simulink model "hyd_hyb_2_int_cont_offline"  (Simulink 8.2)
settings: Solver=ode4  StartTime=0  StopTime=560  FixedStep=0.01  MaxStep=.4  RelTol=1e-8
InitFcn:
  | const_3
values from neighbouring files (symbols this model uses):
  Af = 6.3    [brk_enrg.m]    (also in brk_enrg_1.m)
  BSFC_906_205 = [3.5684 4.3466 5.1668 6.0769 6.988 7.8992 8.8104 9.7336 10.8548 11.9809 13.1112 14.2571 ... (663 elements, 39x17)]    [BSFC_map_906_205.mat]
  Cd = 0.55    [brk_enrg.m]    (also in brk_enrg_1.m)
  den = 1.202    [brk_enrg.m]    (also in brk_enrg_1.m)
  fr = 0.01    [brk_enrg.m]    (also in brk_enrg_1.m)
undefined symbols (not defined in the file or in its folder): clutchRise, down_spd_2, down_spd_3, down_spd_4, down_spd_c, fuel_density, gearshift, I_wheel, Idle_spd_eng_906, M1_hydr, p_v_15, pmax_125, qv_125, Rw, sec_eng_sfc_map, T_max_906, T_min, TC_spd_ratio_max, torque_convertor, Twait, up_spd_1, up_spd_2, up_spd_3, up_spd_c, v_p_10, v_p_15, v_p_5
libraries: fl_lib x43, nesl_utility x30, sdl_lib x14, simulink x4, simulink_need_slupdate x1
(part 2 of 3)

== system hyd_hyb_2_int_cont_offline/hydraulic transmission/controller ==
  T_error : Inport
  Gain : Gain  Gain=1.4
  PID Controller : simulink_need_slupdate/PID Controller  P=0.1  I=10  D=0
  Saturation : Saturate  UpperLimit=125  LowerLimit=-125
  Scope : Scope
      settings: YMin=0  YMax=105  SaveName=ScopeData5
  Transfer Fcn : TransferFcn  Numerator=[1 0]  Denominator=[1 5]
  vg(cm^3/rev) : Outport
  wires:
  T_error/1 -> Gain/1
  Gain/1 -> PID Controller/1
  Saturation/1 -> vg(cm^3/rev)/1
  PID Controller/1 -> Transfer Fcn/1
  Transfer Fcn/1 -> Saturation/1

== system hyd_hyb_2_int_cont_offline/post-transmission torque coupling/Sensor(coupling) ==
  Motion sensor : Subsystem
  Torque sensor : Subsystem
  A : PMIOPort  Port=1  Side=Left
  B : PMIOPort  Port=2  Side=Right
  tag scope: T_coupling=global, w_coupling=global
  wires:
  Torque sensor/1(T) -> [T_coupling]
  Motion sensor/1(W) -> [w_coupling]
  connections:
  B/RConn1 -- Torque sensor/RConn1
  Torque sensor/LConn1 -- Motion sensor/LConn1 -- A/RConn1

== system hyd_hyb_2_int_cont_offline/post-transmission torque coupling/pm gearbox ==
  Ideal Torque Sensor : fl_lib/Mechanical/Mechanical Sensors/Ideal Torque Sensor  w_Log=off  t_Log=off  LocalVarNames=|w|t  LocalVarDescs=|w|t  LocalVarLogging=[0 0]
  Memory : Memory
  PS-Simulink Converter : nesl_utility/PS-Simulink Converter  PhysicalDomain=network_engine_domain  SubClassName=ps_output  LeftPortType=input  RightPortType=output  PseudoPeriodic=off  Frequencies=[]  Unit=N*m  AffineConversion=off
  Simple Gear1 : sdl_lib/Gears/Simple Gear  ratio=1.75  rotation_direction=1  friction_model=1  T_noload=0.1 N*m  T_nom=5 N*m  efficiency_nom=0.8  efficiency=0.8  mu_visc=[ 0 0 ] N*m/(rad/s)  w_thr=0.01 rad/s  LocalVarLogging=[]
  Connection Port : PMIOPort  Tag=PMCPort  Port=1  Side=Left
  Connection Port1 : PMIOPort  Tag=PMCPort  Port=2  Side=Right
  P/M actu_torq(N.m) : Outport
  wires:
  Memory/1 -> P/M actu_torq(N.m)/1
  PS-Simulink Converter/1 -> Memory/1
  connections:
  Simple Gear1/LConn1 -- Connection Port/RConn1
  Simple Gear1/RConn1 -- Ideal Torque Sensor/LConn1
  Ideal Torque Sensor/RConn1 -- Connection Port1/RConn1
  Ideal Torque Sensor/RConn2 -- PS-Simulink Converter/LConn1

== system hyd_hyb_2_int_cont_offline/Engine/Consumption Calc (nmap)1/sfc corrector ==
  main map : Inport
  eng_spd(rpm) : Inport  Port=2
  eng_pow(kw) : Inport  Port=3
  Constant : Constant  Value=Idle_spd_eng_906
  Constant1 : Constant  Value=1000
  Gain : Gain  Gain=-1
  Gain1 : Gain
  Gain2 : Gain
  Product : Product  Inputs=*/  RndMeth=Zero
  Product1 : Product  Inputs=*/  RndMeth=Zero
  Product2 : Product  RndMeth=Zero
  Product3 : Product  RndMeth=Zero
  Scope : Scope  NumInputPorts=2
      settings: YMin=-5~-5  YMax=5~5  SaveName=ScopeData40
  Scope1 : Scope  NumInputPorts=2
      settings: YMin=-5~-5  YMax=5~5  SaveName=ScopeData41
  Scope2 : Scope  NumInputPorts=2
      settings: YMin=-5~-5  YMax=5~5  SaveName=ScopeData42
  Sum : Sum  Inputs=|+-
  Sum1 : Sum  Inputs=|+-
  Sum2 : Sum  Inputs=|+-
  Sum3 : Sum  Inputs=|++
  Switch : Switch  Threshold=1000
  sec_eng_sfc_map (906) : Lookup  InputValues=sec_eng_sfc_map(:,1)  Table=sec_eng_sfc_map(:,2)
  cons(kg/h) : Outport
  wires:
  Gain2/1 -> Product2/1, Scope2/2
  eng_pow(kw)/1 -> sec_eng_sfc_map (906)/1
  Switch/1 -> cons(kg/h)/1
  Sum3/1 -> Switch/3, Scope/2
  Product3/1 -> Sum3/2, Scope1/2
  Product2/1 -> Sum3/1, Scope1/1
  main map/1 -> Product3/1, Switch/1, Scope/1
  sec_eng_sfc_map (906)/1 -> Gain2/1, Scope2/1
  Product1/1 -> Product3/2  "b"
  Gain1/1 -> Product1/1
  Sum2/1 -> Gain1/1
  Product/1 -> Product2/2  "a"
  Sum1/1 -> Product1/2, Product/2
  Constant/1 -> Sum2/2, Sum1/2
  Gain/1 -> Product/1
  Sum/1 -> Gain/1
  Constant1/1 -> Sum1/1, Sum/2
  eng_spd(rpm)/1 -> Switch/2, Sum2/1, Sum/1

== system hyd_hyb_2_int_cont_offline/Engine/Sensor(eng)/Motion sensor ==
  Ideal Rotational Motion Sensor : fl_lib/Mechanical/Mechanical Sensors/Ideal Rotational Motion Sensor  offset=0 rad  w_Log=off  t_Log=off  phi_Log=off  LocalVarNames=|w|t|phi  LocalVarDescs=|w|t|phi  LocalVarLogging=[]
  MRR : fl_lib/Mechanical/Rotational Elements/Mechanical Rotational Reference  t_Log=off  LocalVarNames=|t  LocalVarDescs=|t  LocalVarLogging=[]
  PS-Simulink Converter : nesl_utility/PS-Simulink Converter  PhysicalDomain=network_engine_domain  SubClassName=ps_output  LeftPortType=input  RightPortType=output  PseudoPeriodic=off  Frequencies=[]  Unit=rad/s  AffineConversion=off
  A : PMIOPort  Port=1  Side=Left
  W : Outport
  wires:
  PS-Simulink Converter/1 -> W/1
  connections:
  MRR/LConn1 -- Ideal Rotational Motion Sensor/RConn1
  Ideal Rotational Motion Sensor/RConn2 -- PS-Simulink Converter/LConn1
  A/RConn1 -- Ideal Rotational Motion Sensor/LConn1

== system hyd_hyb_2_int_cont_offline/Engine/Sensor(eng)/Torque sensor ==
  PS2S : nesl_utility/PS-Simulink Converter  PhysicalDomain=network_engine_domain  SubClassName=ps_output  LeftPortType=input  RightPortType=output  PseudoPeriodic=off  Frequencies=[]  Unit=1  AffineConversion=off
  Torque Sensor : fl_lib/Mechanical/Mechanical Sensors/Ideal Torque Sensor  w_Log=off  t_Log=off  LocalVarNames=|w|t  LocalVarDescs=|w|t  LocalVarLogging=[]
  B : PMIOPort  Port=1  Side=Right
  A : PMIOPort  Port=2  Side=Left
  T : Outport
  wires:
  PS2S/1 -> T/1
  connections:
  Torque Sensor/RConn2 -- PS2S/LConn1
  B/RConn1 -- Torque Sensor/RConn1
  A/RConn1 -- Torque Sensor/LConn1

== system hyd_hyb_2_int_cont_offline/Transmission1/Sensor(GB_out)/Motion sensor ==
  Ideal Rotational Motion Sensor : fl_lib/Mechanical/Mechanical Sensors/Ideal Rotational Motion Sensor  offset=0 rad  w_Log=off  t_Log=off  phi_Log=off  LocalVarNames=|w|t|phi  LocalVarDescs=|w|t|phi  LocalVarLogging=[]
  MRR : fl_lib/Mechanical/Rotational Elements/Mechanical Rotational Reference  t_Log=off  LocalVarNames=|t  LocalVarDescs=|t  LocalVarLogging=[]
  PS-Simulink Converter : nesl_utility/PS-Simulink Converter  PhysicalDomain=network_engine_domain  SubClassName=ps_output  LeftPortType=input  RightPortType=output  PseudoPeriodic=off  Frequencies=[]  Unit=rad/s  AffineConversion=off
  A : PMIOPort  Port=1  Side=Left
  W : Outport
  wires:
  PS-Simulink Converter/1 -> W/1
  connections:
  A/RConn1 -- Ideal Rotational Motion Sensor/LConn1
  Ideal Rotational Motion Sensor/RConn2 -- PS-Simulink Converter/LConn1
  MRR/LConn1 -- Ideal Rotational Motion Sensor/RConn1

== system hyd_hyb_2_int_cont_offline/Transmission1/Sensor(GB_out)/Torque sensor ==
  PS2S : nesl_utility/PS-Simulink Converter  PhysicalDomain=network_engine_domain  SubClassName=ps_output  LeftPortType=input  RightPortType=output  PseudoPeriodic=off  Frequencies=[]  Unit=1  AffineConversion=off
  Torque Sensor : fl_lib/Mechanical/Mechanical Sensors/Ideal Torque Sensor  w_Log=off  t_Log=off  LocalVarNames=|w|t  LocalVarDescs=|w|t  LocalVarLogging=[]
  B : PMIOPort  Port=1  Side=Right
  A : PMIOPort  Port=2  Side=Left
  T : Outport
  wires:
  PS2S/1 -> T/1
  connections:
  A/RConn1 -- Torque Sensor/LConn1
  B/RConn1 -- Torque Sensor/RConn1
  Torque Sensor/RConn2 -- PS2S/LConn1

== system hyd_hyb_2_int_cont_offline/Transmission1/Sensor(TC_GB)/Motion sensor ==
  Ideal Rotational Motion Sensor : fl_lib/Mechanical/Mechanical Sensors/Ideal Rotational Motion Sensor  offset=0 rad  w_Log=off  t_Log=off  phi_Log=off  LocalVarNames=|w|t|phi  LocalVarDescs=|w|t|phi  LocalVarLogging=[]
  MRR : fl_lib/Mechanical/Rotational Elements/Mechanical Rotational Reference  t_Log=off  LocalVarNames=|t  LocalVarDescs=|t  LocalVarLogging=[]
  PS-Simulink Converter : nesl_utility/PS-Simulink Converter  PhysicalDomain=network_engine_domain  SubClassName=ps_output  LeftPortType=input  RightPortType=output  PseudoPeriodic=off  Frequencies=[]  Unit=rad/s  AffineConversion=off
  A : PMIOPort  Port=1  Side=Left
  W : Outport
  wires:
  PS-Simulink Converter/1 -> W/1
  connections:
  MRR/LConn1 -- Ideal Rotational Motion Sensor/RConn1
  Ideal Rotational Motion Sensor/RConn2 -- PS-Simulink Converter/LConn1
  A/RConn1 -- Ideal Rotational Motion Sensor/LConn1

== system hyd_hyb_2_int_cont_offline/Transmission1/Sensor(TC_GB)/Torque sensor ==
  PS2S : nesl_utility/PS-Simulink Converter  PhysicalDomain=network_engine_domain  SubClassName=ps_output  LeftPortType=input  RightPortType=output  PseudoPeriodic=off  Frequencies=[]  Unit=1  AffineConversion=off
  Torque Sensor : fl_lib/Mechanical/Mechanical Sensors/Ideal Torque Sensor  w_Log=off  t_Log=off  LocalVarNames=|w|t  LocalVarDescs=|w|t  LocalVarLogging=[]
  B : PMIOPort  Port=1  Side=Right
  A : PMIOPort  Port=2  Side=Left
  T : Outport
  wires:
  PS2S/1 -> T/1
  connections:
  Torque Sensor/RConn2 -- PS2S/LConn1
  B/RConn1 -- Torque Sensor/RConn1
  A/RConn1 -- Torque Sensor/LConn1

== system hyd_hyb_2_int_cont_offline/Transmission1/Torque Convertor/main solver ==
  Add : Sum  Inputs=+-
  Ideal Torque Source1 : fl_lib/Mechanical/Mechanical Sources/Ideal Torque Source  w_Log=off  t_Log=off  LocalVarNames=|w|t  LocalVarDescs=|w|t  LocalVarLogging=[0 0]
  Ideal Torque Source2 : fl_lib/Mechanical/Mechanical Sources/Ideal Torque Source  w_Log=off  t_Log=off  LocalVarNames=|w|t  LocalVarDescs=|w|t  LocalVarLogging=[0 0]
  Mechanical Rotational Reference1 : fl_lib/Mechanical/Rotational Elements/Mechanical Rotational Reference  t_Log=off  LocalVarNames=|t  LocalVarDescs=|t  LocalVarLogging=0
  Sensor(TC_in) : Subsystem
  Sensor(TC_out) : Subsystem
  Simulink-PS Converter1 : nesl_utility/Simulink-PS Converter  PhysicalDomain=network_engine_domain  SubClassName=ps_input  LeftPortType=input  RightPortType=output  PseudoPeriodic=off  Frequencies=[]  NoiseDistribution=none  NoiseParameters=[]  Unit=1  AffineConversion=off  InputFiltering=off  SimscapeFilterOrder=1  InputFilterTimeConstant=0.01  UdotUserProvided=0
  Simulink-PS Converter2 : nesl_utility/Simulink-PS Converter  PhysicalDomain=network_engine_domain  SubClassName=ps_input  LeftPortType=input  RightPortType=output  PseudoPeriodic=off  Frequencies=[]  NoiseDistribution=none  NoiseParameters=[]  Unit=1  AffineConversion=off  InputFiltering=off  SimscapeFilterOrder=1  InputFilterTimeConstant=0.01  UdotUserProvided=0
  Torque generation : Subsystem  AncestorBlock=|
      | driveline/Dynamic
      | Elements/Torque
      | Converter/Torque generation
  T : PMIOPort  Tag=PMCPort  Port=1  Side=Right
  I : PMIOPort  Tag=PMCPort  Port=2  Side=Left
  Turbine torque : Outport
  wires:
  [w_TC_in] -> Torque generation/2(Impeller speed (rad/s))
  Torque generation/1(Turbine torque) -> Turbine torque/1, Simulink-PS Converter1/1
  [w_TC_out] -> Torque generation/1(Turbine speed (rad/s))
  Torque generation/2(Impeller torque) -> Add/1
  [Aux_Trq] -> Add/2
  Add/1 -> Simulink-PS Converter2/1
  connections:
  Ideal Torque Source2/RConn2 -- Mechanical Rotational Reference1/LConn1 -- Ideal Torque Source1/RConn2
  Simulink-PS Converter1/RConn1 -- Ideal Torque Source1/RConn1
  Ideal Torque Source2/RConn1 -- Simulink-PS Converter2/RConn1
  Ideal Torque Source1/LConn1 -- Sensor(TC_out)/LConn1
  Sensor(TC_out)/RConn1 -- T/RConn1
  Ideal Torque Source2/LConn1 -- Sensor(TC_in)/LConn1
  Sensor(TC_in)/RConn1 -- I/RConn1

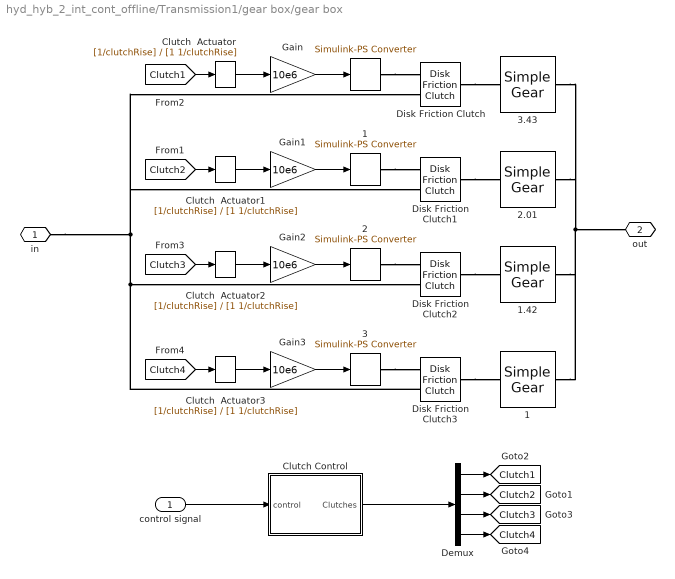
== system hyd_hyb_2_int_cont_offline/Transmission1/gear box/gear box ==
  control signal : Inport
   {,1..3} (4 alike) : nesl_utility/Simulink-PS Converter  PhysicalDomain=network_engine_domain  SubClassName=ps_input  LeftPortType=input  RightPortType=output  PseudoPeriodic=off  Frequencies=[]  NoiseDistribution=none  NoiseParameters=[]  Unit=1  AffineConversion=off  InputFiltering=off  SimscapeFilterOrder=1  InputFilterTimeConstant=0.01  UdotUserProvided=0
  1 : sdl_lib/Gears/Simple Gear  ratio=1  rotation_direction=1  friction_model=1  T_noload=0.1 N*m  T_nom=5 N*m  efficiency_nom=0.8  efficiency=0.8  mu_visc=[ 0 0 ] N*m/(rad/s)  w_thr=0.01 rad/s  LocalVarLogging=[]
  1.42 : sdl_lib/Gears/Simple Gear  ratio=1.42  rotation_direction=1  friction_model=1  T_noload=0.1 N*m  T_nom=5 N*m  efficiency_nom=0.8  efficiency=0.8  mu_visc=[ 0 0 ] N*m/(rad/s)  w_thr=0.01 rad/s  LocalVarLogging=[]
  2.01 : sdl_lib/Gears/Simple Gear  ratio=2.01  rotation_direction=1  friction_model=1  T_noload=0.1 N*m  T_nom=5 N*m  efficiency_nom=0.8  efficiency=0.8  mu_visc=[ 0 0 ] N*m/(rad/s)  w_thr=0.01 rad/s  LocalVarLogging=[]
  3.43 : sdl_lib/Gears/Simple Gear  ratio=3.43  rotation_direction=1  friction_model=1  T_noload=0.1 N*m  T_nom=5 N*m  efficiency_nom=0.8  efficiency=0.8  mu_visc=[ 0 0 ] N*m/(rad/s)  w_thr=0.01 rad/s  LocalVarLogging=[]
  Clutch  Actuator{,1..3} (4 alike) : TransferFcn  Numerator=[1/clutchRise]  Denominator=[1 1/clutchRise]
  Clutch Control : Subsystem
  Demux : Demux
  Disk Friction Clutch : sdl_lib/Clutches/Disk Friction Clutch  geometry_model=1  r_eff=1 m  d_o=150 mm  d_i=100 mm  nS=8  piston_area=0.001 m^2  friction_model=1  mu_coulomb=0.3  mu_w_vector=[ 0 0.1 0.2 0.3 0.4 0.5 1 2 5 10 100 1000 ] rad/s  mu_coulomb_vector=[ 0.29 0.28 0.26 0.22 0.21 0.2 0.2 0.19 0.19 0.19 0.19 0.19 ]  mu_interp_method=1  mu_extrap_method=1  mu_static=0.35  d_f=1  w_tol=0.001 rad/s  pressure_min=100 Pa  mu_visc=0 N*m/(rad/s)  initial_state_locked=0  LocalVarLogging=[]
  Disk Friction Clutch1 : sdl_lib/Clutches/Disk Friction Clutch  geometry_model=1  r_eff=.1 m  d_o=150 mm  d_i=100 mm  nS=8  piston_area=0.001 m^2  friction_model=1  mu_coulomb=0.3  mu_w_vector=[ 0 0.1 0.2 0.3 0.4 0.5 1 2 5 10 100 1000 ] rad/s  mu_coulomb_vector=[ 0.29 0.28 0.26 0.22 0.21 0.2 0.2 0.19 0.19 0.19 0.19 0.19 ]  mu_interp_method=1  mu_extrap_method=1  mu_static=0.35  d_f=1  w_tol=0.001 rad/s  pressure_min=100 Pa  mu_visc=0 N*m/(rad/s)  initial_state_locked=0  LocalVarLogging=[]
  Disk Friction Clutch2 : sdl_lib/Clutches/Disk Friction Clutch  geometry_model=1  r_eff=1 m  d_o=150 mm  d_i=100 mm  nS=8  piston_area=0.001 m^2  friction_model=1  mu_coulomb=0.3  mu_w_vector=[ 0 0.1 0.2 0.3 0.4 0.5 1 2 5 10 100 1000 ] rad/s  mu_coulomb_vector=[ 0.29 0.28 0.26 0.22 0.21 0.2 0.2 0.19 0.19 0.19 0.19 0.19 ]  mu_interp_method=1  mu_extrap_method=1  mu_static=0.35  d_f=1  w_tol=0.001 rad/s  pressure_min=100 Pa  mu_visc=0 N*m/(rad/s)  initial_state_locked=0  LocalVarLogging=[]
  Disk Friction Clutch3 : sdl_lib/Clutches/Disk Friction Clutch  geometry_model=1  r_eff=1 m  d_o=150 mm  d_i=100 mm  nS=8  piston_area=0.001 m^2  friction_model=1  mu_coulomb=0.3  mu_w_vector=[ 0 0.1 0.2 0.3 0.4 0.5 1 2 5 10 100 1000 ] rad/s  mu_coulomb_vector=[ 0.29 0.28 0.26 0.22 0.21 0.2 0.2 0.19 0.19 0.19 0.19 0.19 ]  mu_interp_method=1  mu_extrap_method=1  mu_static=0.35  d_f=1  w_tol=0.001 rad/s  pressure_min=100 Pa  mu_visc=0 N*m/(rad/s)  initial_state_locked=0  LocalVarLogging=[]
  Gain{,1..3} (4 alike) : Gain  Gain=10e6
  in : PMIOPort  Port=1  Side=Left
  out : PMIOPort  Port=2  Side=Right
  tag scope: Clutch1=global, Clutch2=global, Clutch3=global, Clutch4=global
  wires:
  control signal/1 -> Clutch Control/1(control)
  Clutch Control/1(Clutches) -> Demux/1
  Demux/1 -> [Clutch1]
  Demux/2 -> [Clutch2]
  Demux/3 -> [Clutch3]
  Demux/4 -> [Clutch4]
  [Clutch1] -> Clutch  Actuator/1
  [Clutch2] -> Clutch  Actuator1/1
  [Clutch3] -> Clutch  Actuator2/1
  [Clutch4] -> Clutch  Actuator3/1
  Clutch  Actuator/1 -> Gain/1
  Clutch  Actuator1/1 -> Gain1/1
  Clutch  Actuator2/1 -> Gain2/1
  Clutch  Actuator3/1 -> Gain3/1
  Gain/1 -> " "/1
  Gain1/1 -> " 1"/1
  Gain2/1 -> " 2"/1
  Gain3/1 -> " 3"/1
  connections:
  Disk Friction Clutch3/LConn2 -- in/RConn1 -- Disk Friction Clutch/LConn2 -- Disk Friction Clutch1/LConn2 -- Disk Friction Clutch2/LConn2
  1.42/RConn1 -- 3.43/RConn1 -- 1/RConn1 -- 2.01/RConn1 -- out/RConn1
  " "/RConn1 -- Disk Friction Clutch/LConn1
  " 1"/RConn1 -- Disk Friction Clutch1/LConn1
  " 2"/RConn1 -- Disk Friction Clutch2/LConn1
  " 3"/RConn1 -- Disk Friction Clutch3/LConn1
  Disk Friction Clutch/RConn1 -- 3.43/LConn1
  Disk Friction Clutch1/RConn1 -- 2.01/LConn1
  Disk Friction Clutch2/RConn1 -- 1.42/LConn1
  Disk Friction Clutch3/RConn1 -- 1/LConn1

== system hyd_hyb_2_int_cont_offline/Vehicle Dynamic/Resistance Load/Aerodynamic Force ==
  note: Fa
  note: Fr
  V : Inport
  0.5*Cd*den*Ar : Gain  Gain=0.5*Cd*den*Af  SaturateOnIntegerOverflow=on  OutDataTypeStr=Inherit: Same as input  ParamDataTypeStr=Inherit: Same as input
  Constant1 : Constant  Value=0
  V^2 : Math  Operator=square  SaturateOnIntegerOverflow=on
  check  v=0 : Switch  Criteria=u2 > Threshold
  Fa : Outport
  wires:
  V^2/1 -> 0.5*Cd*den*Ar/1
  V/1 -> V^2/1, check  v=0/2
  Constant1/1 -> check  v=0/3
  0.5*Cd*den*Ar/1 -> check  v=0/1
  check  v=0/1 -> Fa/1

== system hyd_hyb_2_int_cont_offline/Vehicle Dynamic/Resistance Load/Grade Force ==
  note: Fr
  slope : Inport
  V : Inport  Port=2
  accum_mass : Inport  Port=3
  Constant : Constant  Value=9.81
  Constant1 : Constant  Value=0
  Constant2 : Constant  Value=M1_hydr
  Product : Product  SaturateOnIntegerOverflow=on  RndMeth=Zero  InputSameDT=on  OutDataTypeStr=Inherit: Same as first input
  Product1 : Product  RndMeth=Zero
  Sum : Sum  Inputs=|++
  check  v=0 : Switch  Criteria=u2 > Threshold
  degree 2 rad : Gain  Gain=pi/180  SaturateOnIntegerOverflow=on  OutDataTypeStr=Inherit: Same as input  ParamDataTypeStr=Inherit: Same as input
  sin(teta) : Trigonometry
  Fg : Outport
  wires:
  slope/1 -> degree 2 rad/1
  sin(teta)/1 -> Product/2
  degree 2 rad/1 -> sin(teta)/1
  V/1 -> check  v=0/2
  Constant1/1 -> check  v=0/3
  check  v=0/1 -> Fg/1
  Product/1 -> check  v=0/1
  accum_mass/1 -> Sum/1
  Constant2/1 -> Sum/2
  Constant/1 -> Product1/1
  Sum/1 -> Product1/2
  Product1/1 -> Product/1

== system hyd_hyb_2_int_cont_offline/Vehicle Dynamic/Resistance Load/Rolling Force ==
  note: Fr
  V : Inport
  accum_mass : Inport  Port=2
  Constant : Constant  Value=9.81
  Constant1 : Constant  Value=0
  Constant2 : Constant  Value=M1_hydr
  Product : Product  RndMeth=Zero
  Sum : Sum  Inputs=|++
  check  v=0 : Switch  Criteria=u2 > Threshold
  fr : Gain  Gain=fr  SaturateOnIntegerOverflow=on  OutDataTypeStr=Inherit: Same as input  ParamDataTypeStr=Inherit: Same as input
  Fr : Outport
  wires:
  V/1 -> check  v=0/2
  Constant1/1 -> check  v=0/3
  fr/1 -> check  v=0/1
  check  v=0/1 -> Fr/1
  accum_mass/1 -> Sum/1
  Constant2/1 -> Sum/2
  Constant/1 -> Product/1
  Sum/1 -> Product/2
  Product/1 -> fr/1

== system hyd_hyb_2_int_cont_offline/Vehicle Dynamic/Sensor(follower)/Motion sensor ==
  Ideal Rotational Motion Sensor : fl_lib/Mechanical/Mechanical Sensors/Ideal Rotational Motion Sensor  offset=0 rad  w_Log=off  t_Log=off  phi_Log=off  LocalVarNames=|w|t|phi  LocalVarDescs=|w|t|phi  LocalVarLogging=[]
  MRR : fl_lib/Mechanical/Rotational Elements/Mechanical Rotational Reference  t_Log=off  LocalVarNames=|t  LocalVarDescs=|t  LocalVarLogging=[]
  PS-Simulink Converter : nesl_utility/PS-Simulink Converter  PhysicalDomain=network_engine_domain  SubClassName=ps_output  LeftPortType=input  RightPortType=output  PseudoPeriodic=off  Frequencies=[]  Unit=rad/s  AffineConversion=off
  A : PMIOPort  Port=1  Side=Left
  W : Outport
  wires:
  PS-Simulink Converter/1 -> W/1
  connections:
  MRR/LConn1 -- Ideal Rotational Motion Sensor/RConn1
  Ideal Rotational Motion Sensor/RConn2 -- PS-Simulink Converter/LConn1
  A/RConn1 -- Ideal Rotational Motion Sensor/LConn1

== system hyd_hyb_2_int_cont_offline/Vehicle Dynamic/Sensor(follower)/Torque sensor ==
  PS2S : nesl_utility/PS-Simulink Converter  PhysicalDomain=network_engine_domain  SubClassName=ps_output  LeftPortType=input  RightPortType=output  PseudoPeriodic=off  Frequencies=[]  Unit=1  AffineConversion=off
  Torque Sensor : fl_lib/Mechanical/Mechanical Sensors/Ideal Torque Sensor  w_Log=off  t_Log=off  LocalVarNames=|w|t  LocalVarDescs=|w|t  LocalVarLogging=[]
  B : PMIOPort  Port=1  Side=Right
  A : PMIOPort  Port=2  Side=Left
  T : Outport
  wires:
  PS2S/1 -> T/1
  connections:
  Torque Sensor/RConn2 -- PS2S/LConn1
  B/RConn1 -- Torque Sensor/RConn1
  A/RConn1 -- Torque Sensor/LConn1

== system hyd_hyb_2_int_cont_offline/hydraulic transmission/PM_hydraulic_machine /base variables ==
  p_accum : Inport
  n(rpm) : Inport  Port=2
  vg(cm^3/rev) : Inport  Port=3
  SOC_min(%) : Inport  Port=4
  SOC : Inport  Port=5
  Add : Sum  Inputs=+-
  Constant : Constant  Value=0.000001
  Scope2 : Scope
      settings: TimeRange=2  YMin=181  YMax=194  SaveName=ScopeData49
  Switch : Switch  Criteria=u2 ~= 0
  air pressure : Constant  Value=1.01
  vg : Outport
  delta_p : Outport  Port=2
  n : Outport  Port=3
  SOC1 : Outport  Port=4
  SOC_min : Outport  Port=5
  wires:
  p_accum/1 -> Add/1
  air pressure/1 -> Add/2
  vg(cm^3/rev)/1 -> Switch/2, Switch/1
  Constant/1 -> Switch/3
  Switch/1 -> vg/1
  Add/1 -> delta_p/1, Scope2/1
  n(rpm)/1 -> n/1
  SOC/1 -> SOC1/1
  SOC_min(%)/1 -> SOC_min/1

== system hyd_hyb_2_int_cont_offline/hydraulic transmission/PM_hydraulic_machine /eta estimator ==
  qv : Inport
  delta_p : Inport  Port=2
  Pmax : Inport  Port=3
  vg : Inport  Port=4
  n : Inport  Port=5
  Saturation : Saturate  UpperLimit=1  LowerLimit=0.75
  eta_mh2 : Product  Inputs=*/
  eta_t : Subsystem
  eta_v : Subsystem
  eta_mh : Outport
  wires:
  eta_t/1(eta_t) -> eta_mh2/1
  eta_v/1(eta_v) -> eta_mh2/2
  eta_mh2/1 -> Saturation/1
  Saturation/1 -> eta_mh/1
  qv/1 -> eta_t/1(qv), eta_v/1(qv)
  delta_p/1 -> eta_t/2(delta_p)
  Pmax/1 -> eta_t/3(Pmax)
  vg/1 -> eta_v/2(vg)
  n/1 -> eta_v/3(n)

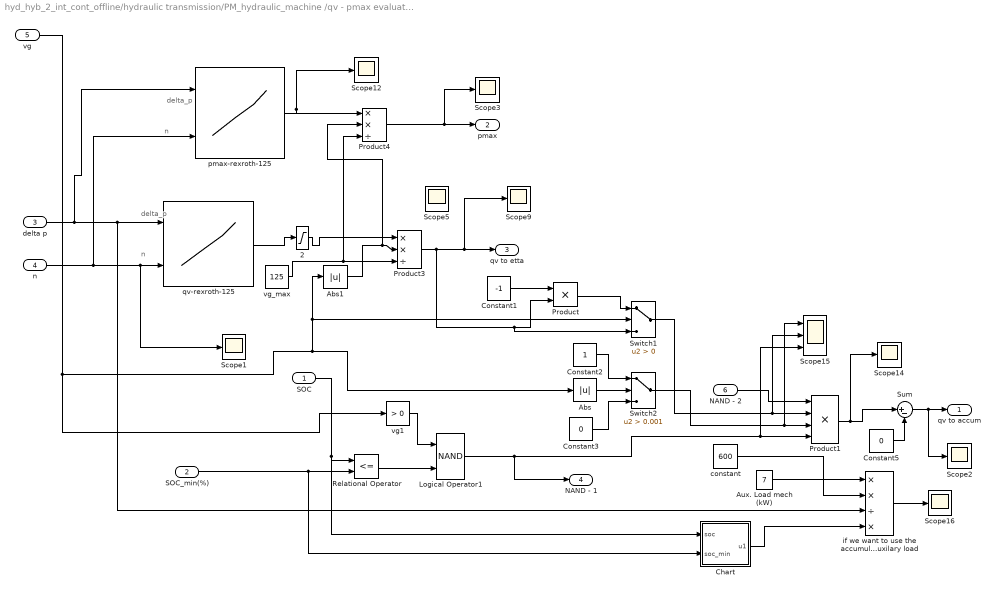
== system hyd_hyb_2_int_cont_offline/hydraulic transmission/PM_hydraulic_machine /qv - pmax evaluation ==
  note: delta_p
  note: delta_p
  note: n
  note: n
  SOC : Inport
  SOC_min(%) : Inport  Port=2
  delta p : Inport  Port=3
  n : Inport  Port=4
  vg : Inport  Port=5
  NAND - 2 : Inport  Port=6
  2 : Saturate  UpperLimit=inf  LowerLimit=0
  Abs : Abs
  Abs1 : Abs
  Aux. Load mech (kW) : Constant  Value=7
  Chart : Stateflow chart  TreatAsAtomicUnit=on
  Constant1 : Constant  Value=-1
  Constant2 : Constant
  Constant3 : Constant  Value=0
  Constant5 : Constant  Value=0
  Logical Operator1 : Logic  Operator=NAND  AllPortsSameDT=off  OutDataTypeStr=boolean
  Product : Product  RndMeth=Zero
  Product1 : Product  Inputs=4  RndMeth=Zero
  Product3 : Product  Inputs=**/  RndMeth=Zero
  Product4 : Product  Inputs=**/  RndMeth=Zero
  Relational Operator : RelationalOperator  Operator=<=  OutDataTypeStr=boolean
  Scope{1..3,5,9,12,14,16} (8 alike) : Scope
      Scope1 settings: YMin=660  YMax=880  SaveName=ScopeData79
      Scope12 settings: YMin=-200  YMax=350  SaveName=ScopeData81
      Scope14 settings: TimeRange=2  YMin=5.391  YMax=5.413  SaveName=ScopeData54
      Scope16 settings: YMin=5.45  YMax=6.1  SaveName=ScopeData96
      Scope2 settings: YMin=-15  YMax=85  SaveName=ScopeData85
      Scope3 settings: YMin=-200  YMax=350  SaveName=ScopeData87
      Scope5 settings: TimeRange=2  YMin=-200  YMax=350  SaveName=ScopeData82
      Scope9 settings: YMin=-200  YMax=350  SaveName=ScopeData86
  Scope15 : Scope  NumInputPorts=3
      settings: YMin=-200~-5~-5  YMax=350~5~5  SaveName=ScopeData72
  Sum : Sum  Inputs=|+-
  Switch1 : Switch  Criteria=u2 > Threshold
  Switch2 : Switch  Criteria=u2 > Threshold  Threshold=0.001
  constant : Constant  Value=600
  if we want to use the accumulator for auxilary load : Product  Inputs=**/*  RndMeth=Zero
  pmax-rexroth-125 : Lookup2D  RowIndex=[0:10:350]  ColumnIndex=[800:100:1800]  Table=pmax_125
  qv-rexroth-125 : Lookup2D  RowIndex=[0:10:350]  ColumnIndex=[800:100:1800]  Table=qv_125
  vg1 : simulink/Logic and Bit Operations/Compare To Constant  relop=>  const=0  OutDataTypeStr=uint8  ZeroCross=off
  vg_max : Constant  Value=125
  qv to accum : Outport
  pmax : Outport  Port=2
  qv to etta : Outport  Port=3
  NAND - 1 : Outport  Port=4
  wires:
  pmax-rexroth-125/1 -> Scope12/1, Product4/1
  delta p/1 -> qv-rexroth-125/1, if we want to use the accumulator for auxilary load/3, pmax-rexroth-125/1
  n/1 -> pmax-rexroth-125/2, qv-rexroth-125/2, Scope1/1
  vg/1 -> vg1/1, Abs/1, Abs1/1, Switch1/2
  qv-rexroth-125/1 -> 2/1
  SOC/1 -> Relational Operator/1, Chart/1(soc)
  SOC_min(%)/1 -> Relational Operator/2, Chart/2(soc_min)
  Relational Operator/1 -> Logical Operator1/2
  vg1/1 -> Logical Operator1/1
  Abs1/1 -> Product3/2, Product4/2
  Product4/1 -> pmax/1, Scope3/1
  vg_max/1 -> Product3/3, Product4/3
  2/1 -> Product3/1
  Product/1 -> Switch1/1
  Constant1/1 -> Product/1
  Switch1/1 -> Product1/2, Scope15/2
  Abs/1 -> Switch2/2
  Constant2/1 -> Switch2/1
  Constant3/1 -> Switch2/3
  Switch2/1 -> Product1/3, Scope15/1
  Sum/1 -> qv to accum/1, Scope2/1
  Product1/1 -> Sum/1, Scope14/1
  Aux. Load mech (kW)/1 -> if we want to use the accumulator for auxilary load/1
  constant/1 -> if we want to use the accumulator for auxilary load/2
  Product3/1 -> Product/2, Switch1/3, qv to etta/1, Scope9/1
  Logical Operator1/1 -> NAND - 1/1, Product1/4, Scope15/3
  NAND - 2/1 -> Product1/1
  if we want to use the accumulator for auxilary load/1 -> Scope16/1
  Chart/1(u1) -> if we want to use the accumulator for auxilary load/4
  Constant5/1 -> Sum/2

== system hyd_hyb_2_int_cont_offline/hydraulic transmission/PM_hydraulic_machine /torque estimator ==
  vg : Inport
  eta_mh : Inport  Port=2
  delta_p : Inport  Port=3
  n : Inport  Port=4
  SOC : Inport  Port=5
  NAND_1 : Inport  Port=6
  Constant : Constant  Value=20*pi
  Constant1 : Constant  Value=0.9
  Logical Operator : Logic  Operator=NAND  AllPortsSameDT=off  OutDataTypeStr=boolean
  Product2 : Product  Inputs=3  RndMeth=Zero
  Scope : Scope
      settings: YMin=-100  YMax=300  SaveName=ScopeData6
  Scope2 : Scope  NumInputPorts=3
      settings: YMin=-20~167.7~0.75  YMax=75~170~0.86  SaveName=ScopeData8
  Switch1 : Switch  Criteria=u2 > Threshold
  Switch2 : Switch  Criteria=u2 > Threshold  Threshold=400
  motor : Product  Inputs=***/
  pump : Product  Inputs=**//
  soc : simulink/Logic and Bit Operations/Compare To Constant  relop=>=  const=100  OutDataTypeStr=uint8  ZeroCross=off
  vg1 : simulink/Logic and Bit Operations/Compare To Constant  relop=<  const=0  OutDataTypeStr=uint8  ZeroCross=off
  T(N.m) : Outport
  NAND_2 : Outport  Port=2
  wires:
  vg/1 -> pump/1, motor/1, Scope2/1, Switch1/2, vg1/1
  delta_p/1 -> pump/2, motor/2, Scope2/2
  Constant/1 -> pump/4, motor/4
  pump/1 -> Switch1/3
  motor/1 -> Switch1/1
  n/1 -> Switch2/2
  eta_mh/1 -> Switch2/1
  Constant1/1 -> Switch2/3
  Switch2/1 -> pump/3, motor/3, Scope2/3
  Logical Operator/1 -> Product2/2, NAND_2/1
  vg1/1 -> Logical Operator/1
  soc/1 -> Logical Operator/2
  Product2/1 -> T(N.m)/1, Scope/1
  Switch1/1 -> Product2/1
  NAND_1/1 -> Product2/3
  SOC/1 -> soc/1

== system hyd_hyb_2_int_cont_offline/hydraulic transmission/Sensor(PM)/Motion sensor ==
  Ideal Rotational Motion Sensor : fl_lib/Mechanical/Mechanical Sensors/Ideal Rotational Motion Sensor  offset=0 rad  w_Log=off  t_Log=off  phi_Log=off  LocalVarNames=|w|t|phi  LocalVarDescs=|w|t|phi  LocalVarLogging=[]
  MRR : fl_lib/Mechanical/Rotational Elements/Mechanical Rotational Reference  t_Log=off  LocalVarNames=|t  LocalVarDescs=|t  LocalVarLogging=[]
  PS-Simulink Converter : nesl_utility/PS-Simulink Converter  PhysicalDomain=network_engine_domain  SubClassName=ps_output  LeftPortType=input  RightPortType=output  PseudoPeriodic=off  Frequencies=[]  Unit=rad/s  AffineConversion=off
  A : PMIOPort  Port=1  Side=Left
  W : Outport
  wires:
  PS-Simulink Converter/1 -> W/1
  connections:
  MRR/LConn1 -- Ideal Rotational Motion Sensor/RConn1
  Ideal Rotational Motion Sensor/RConn2 -- PS-Simulink Converter/LConn1
  A/RConn1 -- Ideal Rotational Motion Sensor/LConn1

== system hyd_hyb_2_int_cont_offline/hydraulic transmission/Sensor(PM)/Torque sensor ==
  PS2S : nesl_utility/PS-Simulink Converter  PhysicalDomain=network_engine_domain  SubClassName=ps_output  LeftPortType=input  RightPortType=output  PseudoPeriodic=off  Frequencies=[]  Unit=1  AffineConversion=off
  Torque Sensor : fl_lib/Mechanical/Mechanical Sensors/Ideal Torque Sensor  w_Log=off  t_Log=off  LocalVarNames=|w|t  LocalVarDescs=|w|t  LocalVarLogging=[]
  B : PMIOPort  Port=1  Side=Right
  A : PMIOPort  Port=2  Side=Left
  T : Outport
  wires:
  PS2S/1 -> T/1
  connections:
  Torque Sensor/RConn2 -- PS2S/LConn1
  B/RConn1 -- Torque Sensor/RConn1
  A/RConn1 -- Torque Sensor/LConn1

== system hyd_hyb_2_int_cont_offline/hydraulic transmission/accumulator/SOC estimator ==
  max_vol : Inport
  v_x : Inport  Port=2
  min_vol : Inport  Port=3
  Divide1 : Product  Inputs=*/
  Divide3 : Product  Inputs=*/
  Gain : Gain  Gain=100
  Gain5 : Gain  Gain=100
  Scope1 : Scope
      settings: YMin=11.5531  YMax=12.7693  SaveName=ScopeData6
  Scope6 : Scope
      settings: SaveName=ScopeData4
  SOC(%) : Outport
  SOC_min(%) : Outport  Port=2
  wires:
  Divide1/1 -> Gain/1
  Gain/1 -> SOC(%)/1, Scope6/1
  Gain5/1 -> SOC_min(%)/1, Scope1/1
  Divide3/1 -> Gain5/1
  min_vol/1 -> Divide3/1
  max_vol/1 -> Divide3/2, Divide1/2
  v_x/1 -> Divide1/1

== system hyd_hyb_2_int_cont_offline/hydraulic transmission/accumulator/accum_pres & vol estimator ==
  v_x : Inport
  init_SOC : Inport  Port=2
  max_vol : Inport  Port=3
  accum_num : Inport  Port=4
  pre_ch_press(psi) : Inport  Port=5
  accum_type : Inport  Port=6
  Gain : Gain  Gain=61.02
  Gain1 : Gain  Gain=0.0689
  Product1 : Product  Inputs=3  RndMeth=Zero
  Scope1 : Scope
  Scope3 : Scope  NumInputPorts=3
      settings: YMin=-5~-5~-5  YMax=5~5~5  SaveName=ScopeData2
  Scope4 : Scope
      settings: YMin=2500  YMax=2825  SaveName=ScopeData103
  Scope5 : Scope
      settings: YMin=140.5  YMax=147  SaveName=ScopeData104
  Switch : Switch  Criteria=u2 > Threshold  Threshold=12
  Switch1 : Switch  Criteria=u2 > Threshold  Threshold=7
  rexroth-10 : Lookup_n-D  BreakpointsForDimension1=[0:33.8889:1559]  BreakpointsForDimension2=[1000,1400,2000]  Table=p_v_15  InputSameDT=on
  rexroth-15 : Lookup_n-D  BreakpointsForDimension1=[0,50,100,150,200,250,300,350,400,450,500,550,600,650,700,750,800,850,900,950,1000,1050,1100,1150,1200,1250,1300,1350,1400,1450,1500,1550,1600,1650,1700,1750,1800,1850,1900,1950,2000,2050,2100,2150,2200,2250,2300]  BreakpointsForDimension2=[1000,1400,2000]  Table=p_v_15  InputSameDT=on
  rexroth-5 : Lookup_n-D  BreakpointsForDimension1=[0:17.33:814]  BreakpointsForDimension2=[1000,1400,2000]  Table=p_v_15  InputSameDT=on
  accum_pres(bar) : Outport
  accum_init_vol(lit) : Outport  Port=2
  wires:
  Product1/1 -> accum_init_vol(lit)/1, Scope1/1
  init_SOC/1 -> Product1/1, Scope3/1
  max_vol/1 -> Product1/2, Scope3/2
  accum_num/1 -> Product1/3, Scope3/3
  pre_ch_press(psi)/1 -> rexroth-15/2, rexroth-10/2, rexroth-5/2
  v_x/1 -> Gain/1
  Gain/1 -> rexroth-15/1, rexroth-10/1, rexroth-5/1
  Gain1/1 -> Scope5/1, accum_pres(bar)/1
  accum_type/1 -> Switch/2, Switch1/2
  rexroth-15/1 -> Switch/1
  Switch1/1 -> Switch/3
  rexroth-10/1 -> Switch1/1
  rexroth-5/1 -> Switch1/3
  Switch/1 -> Gain1/1, Scope4/1

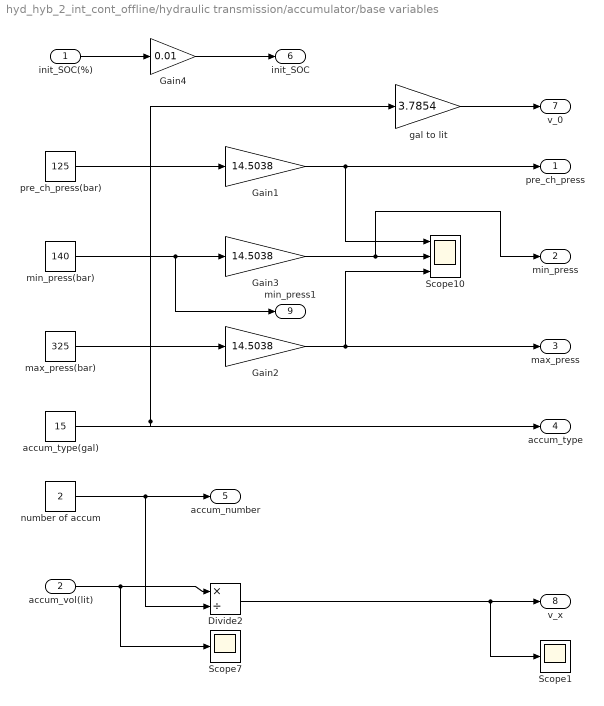
== system hyd_hyb_2_int_cont_offline/hydraulic transmission/accumulator/base variables ==
  init_SOC(%) : Inport
  accum_vol(lit) : Inport  Port=2
  Divide2 : Product  Inputs=*/
  Gain1 : Gain  Gain=14.5038
  Gain2 : Gain  Gain=14.5038
  Gain3 : Gain  Gain=14.5038
  Gain4 : Gain  Gain=0.01
  Scope1 : Scope
      settings: YMin=3138.26  YMax=3138.33  SaveName=ScopeData5
  Scope10 : Scope  NumInputPorts=3
      settings: YMin=1929~2204.58~4753.62  YMax=2132.06~2436.64~5254
  Scope7 : Scope
      settings: YMin=3138.26  YMax=3138.33  SaveName=ScopeData3
  accum_type(gal) : Constant  Value=15
  gal to lit : Gain  Gain=3.7854
  max_press(bar) : Constant  Value=325
  min_press(bar) : Constant  Value=140
  number of accum : Constant  Value=2
  pre_ch_press(bar) : Constant  Value=125
  pre_ch_press : Outport
  min_press : Outport  Port=2
  max_press : Outport  Port=3
  accum_type : Outport  Port=4
  accum_number : Outport  Port=5
  init_SOC : Outport  Port=6
  v_0 : Outport  Port=7
  v_x : Outport  Port=8
  min_press1 : Outport  Port=9
  wires:
  accum_type(gal)/1 -> gal to lit/1, accum_type/1
  init_SOC(%)/1 -> Gain4/1
  pre_ch_press(bar)/1 -> Gain1/1
  min_press(bar)/1 -> Gain3/1, min_press1/1
  max_press(bar)/1 -> Gain2/1
  Gain1/1 -> Scope10/1, pre_ch_press/1
  Gain3/1 -> Scope10/2, min_press/1
  Gain2/1 -> Scope10/3, max_press/1
  Gain4/1 -> init_SOC/1
  number of accum/1 -> accum_number/1, Divide2/2
  accum_vol(lit)/1 -> Divide2/1, Scope7/1
  gal to lit/1 -> v_0/1
  Divide2/1 -> v_x/1, Scope1/1

== system hyd_hyb_2_int_cont_offline/hydraulic transmission/accumulator/max - min volume estimator ==
  min_press : Inport
  max_press : Inport  Port=2
  pre_c_press : Inport  Port=3
  accum_size : Inport  Port=4
  accum_num : Inport  Port=5
  Add : Sum  Inputs=+++
  Add1 : Sum  Inputs=+++
  Add2 : Sum  Inputs=+++
  If : If  IfExpression=u1 == 5  ShowElse=off
  If1 : If  IfExpression=u1 == 10  ShowElse=off
  If2 : If  IfExpression=u1 == 15  ShowElse=off
  Product : Product  RndMeth=Zero
  Scope1 : Scope  NumInputPorts=3
      settings: YMin=95~-5~-5  YMax=105~5~5  SaveName=ScopeData101
  Scope4 : Scope  NumInputPorts=3
      settings: YMin=-1~-1~22.8383  YMax=1~1~25.2423  SaveName=ScopeData7
  Scope5 : Scope  NumInputPorts=3
      settings: YMin=-1~-1~4.5076  YMax=1~1~4.98208  SaveName=ScopeData8
  for 10 gal accumulator : Subsystem  TreatAsAtomicUnit=on
  for 15 gal accumulator1 : Subsystem  TreatAsAtomicUnit=on
  for 5 gal accumulator : Subsystem  TreatAsAtomicUnit=on
  min_vol : Outport
  max_vol : Outport  Port=2
  accum_dry_mass ( kg ) : Outport  Port=3
  wires:
  for 5 gal accumulator/1(min_vol(lit)) -> Add/1, Scope5/1
  for 10 gal accumulator/1(min_vol(lit)) -> Add/2, Scope5/2
  for 15 gal accumulator1/1(min_vol(lit)) -> Scope5/3, Add/3
  for 5 gal accumulator/2(max_vol(lit)) -> Add1/1, Scope4/1
  for 10 gal accumulator/2(max_vol(lit)) -> Add1/2, Scope4/2
  for 15 gal accumulator1/2(max_vol(lit)) -> Add1/3, Scope4/3
  If/1 -> for 5 gal accumulator/Action
  If2/1 -> for 15 gal accumulator1/Action
  Add/1 -> min_vol/1
  Add1/1 -> max_vol/1
  min_press/1 -> for 5 gal accumulator/1(min_press(psi)), for 10 gal accumulator/1(min_press(psi)), for 15 gal accumulator1/1(min_press(psi))
  max_press/1 -> for 5 gal accumulator/2(max_press(psi)), for 10 gal accumulator/2(max_press(psi)), for 15 gal accumulator1/2(max_press(psi))
  pre_c_press/1 -> for 5 gal accumulator/3(pre_ch_press(psi)), for 10 gal accumulator/3(pre_ch_press(psi)), for 15 gal accumulator1/3(pre_ch_press(psi))
  accum_size/1 -> If1/1, If/1, If2/1
  If1/1 -> for 10 gal accumulator/Action
  for 5 gal accumulator/3(accum_dry_mass ( kg )) -> Add2/1, Scope1/1
  for 10 gal accumulator/3(accum_dry_mass ( kg )) -> Add2/2, Scope1/2
  for 15 gal accumulator1/3(accum_dry_mass ( kg )) -> Add2/3, Scope1/3
  Add2/1 -> Product/1
  accum_num/1 -> Product/2
  Product/1 -> accum_dry_mass ( kg )/1

== system hyd_hyb_2_int_cont_offline/post-transmission torque coupling/Sensor(coupling)/Motion sensor ==
  Ideal Rotational Motion Sensor : fl_lib/Mechanical/Mechanical Sensors/Ideal Rotational Motion Sensor  offset=0 rad  w_Log=off  t_Log=off  phi_Log=off  LocalVarNames=|w|t|phi  LocalVarDescs=|w|t|phi  LocalVarLogging=[]
  MRR : fl_lib/Mechanical/Rotational Elements/Mechanical Rotational Reference  t_Log=off  LocalVarNames=|t  LocalVarDescs=|t  LocalVarLogging=[]
  PS-Simulink Converter : nesl_utility/PS-Simulink Converter  PhysicalDomain=network_engine_domain  SubClassName=ps_output  LeftPortType=input  RightPortType=output  PseudoPeriodic=off  Frequencies=[]  Unit=rad/s  AffineConversion=off
  A : PMIOPort  Port=1  Side=Left
  W : Outport
  wires:
  PS-Simulink Converter/1 -> W/1
  connections:
  MRR/LConn1 -- Ideal Rotational Motion Sensor/RConn1
  Ideal Rotational Motion Sensor/RConn2 -- PS-Simulink Converter/LConn1
  A/RConn1 -- Ideal Rotational Motion Sensor/LConn1

== system hyd_hyb_2_int_cont_offline/post-transmission torque coupling/Sensor(coupling)/Torque sensor ==
  PS2S : nesl_utility/PS-Simulink Converter  PhysicalDomain=network_engine_domain  SubClassName=ps_output  LeftPortType=input  RightPortType=output  PseudoPeriodic=off  Frequencies=[]  Unit=1  AffineConversion=off
  Torque Sensor : fl_lib/Mechanical/Mechanical Sensors/Ideal Torque Sensor  w_Log=off  t_Log=off  LocalVarNames=|w|t  LocalVarDescs=|w|t  LocalVarLogging=[]
  B : PMIOPort  Port=1  Side=Right
  A : PMIOPort  Port=2  Side=Left
  T : Outport
  wires:
  PS2S/1 -> T/1
  connections:
  Torque Sensor/RConn2 -- PS2S/LConn1
  B/RConn1 -- Torque Sensor/RConn1
  A/RConn1 -- Torque Sensor/LConn1

== system hyd_hyb_2_int_cont_offline/Transmission1/Torque Convertor/main solver/Sensor(TC_in) ==
  Motion sensor : Subsystem
  Torque sensor : Subsystem
  A : PMIOPort  Port=1  Side=Left
  B : PMIOPort  Port=2  Side=Right
  tag scope: T_TC_in=global, w_TC_in=global
  wires:
  Motion sensor/1(W) -> [w_TC_in]
  Torque sensor/1(T) -> [T_TC_in]
  connections:
  A/RConn1 -- Motion sensor/LConn1 -- Torque sensor/LConn1
  B/RConn1 -- Torque sensor/RConn1

== system hyd_hyb_2_int_cont_offline/Transmission1/Torque Convertor/main solver/Sensor(TC_out) ==
  Motion sensor : Subsystem
  Torque sensor : Subsystem
  A : PMIOPort  Port=1  Side=Left
  B : PMIOPort  Port=2  Side=Right
  tag scope: T_TC_out=global, w_TC_out=global
  wires:
  Torque sensor/1(T) -> [T_TC_out]
  Motion sensor/1(W) -> [w_TC_out]
  connections:
  B/RConn1 -- Torque sensor/RConn1
  Torque sensor/LConn1 -- Motion sensor/LConn1 -- A/RConn1

== system hyd_hyb_2_int_cont_offline/Transmission1/Torque Convertor/main solver/Torque generation ==
  note: TORQUE CONVERTER
  note: Not motoring mode is neglected
  Turbine speed (rad/s) : Inport
  Impeller speed (rad/s) : Inport  Port=2
  4 : Product  Inputs=/*  SaturateOnIntegerOverflow=on  RndMeth=Zero  InputSameDT=on  OutDataTypeStr=Inherit: Same as first input
  Constant1 : Constant
  Constant2 : Constant  Value=eps
  Constant6 : Constant  Value=TC_spd_ratio_max
  Gain1 : Gain  Gain=-1  SaturateOnIntegerOverflow=on  OutDataTypeStr=Inherit: Same as input  ParamDataTypeStr=Inherit: Same as input
  Math Function1 : Math  Operator=square  SaturateOnIntegerOverflow=on
  Memory : Memory
  Memory1 : Memory
  MinMax2 : MinMax  Function=max  Inputs=2  ZeroCross=off
  Mu : Lookup  InputValues=torque_convertor(:,1)  Table=torque_convertor(:,2)  SaturateOnIntegerOverflow=on
  Ref_spd (rpm) : Constant  Value=1000
  T1 : Scope  NumInputPorts=2
      settings: YMin=75~-5  YMax=165~5  SaveName=ScopeData19
  T_i : Product  Inputs=**  SaturateOnIntegerOverflow=on  RndMeth=Zero  InputSameDT=on  OutDataTypeStr=Inherit: Same as first input
  T_t : Product  Inputs=**  SaturateOnIntegerOverflow=on  RndMeth=Zero  InputSameDT=on  OutDataTypeStr=Inherit: Same as first input
  check pump spd=0 : Switch  Threshold=0.1
  check turb spd=0 : Switch  Threshold=0.1
  pump T : Lookup  InputValues=torque_convertor(:,1)  Table=torque_convertor(:,3)  SaturateOnIntegerOverflow=on
  rad/s 2 rpm : Gain  Gain=60/(2*pi)
  speed ratio : Product  Inputs=/*  SaturateOnIntegerOverflow=on  RndMeth=Zero  InputSameDT=on  OutDataTypeStr=Inherit: Same as first input
  Turbine torque : Outport
  Impeller torque : Outport  Port=2
  wires:
  Constant2/1 -> MinMax2/2
  MinMax2/1 -> speed ratio/1
  Impeller speed (rad/s)/1 -> MinMax2/1, check pump spd=0/2, rad/s 2 rpm/1
  Turbine speed (rad/s)/1 -> check turb spd=0/2, speed ratio/2
  speed ratio/1 -> check pump spd=0/1
  Constant1/1 -> check turb spd=0/3
  Constant6/1 -> check turb spd=0/1
  check turb spd=0/1 -> check pump spd=0/3
  check pump spd=0/1 -> Mu/1, pump T/1
  Ref_spd (rpm)/1 -> 4/1
  rad/s 2 rpm/1 -> 4/2
  4/1 -> Math Function1/1
  pump T/1 -> T_i/1
  Math Function1/1 -> T_i/2
  T_i/1 -> T_t/2, Gain1/1
  Gain1/1 -> Memory1/1
  Mu/1 -> T_t/1
  T_t/1 -> Memory/1
  Memory/1 -> Turbine torque/1
  Memory1/1 -> Impeller torque/1

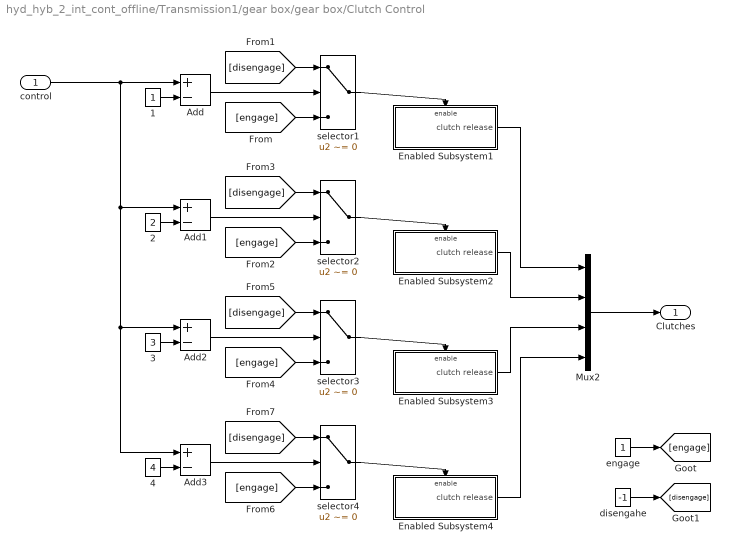
== system hyd_hyb_2_int_cont_offline/Transmission1/gear box/gear box/Clutch Control ==
  control : Inport
  1 : Constant
  2 : Constant  Value=2
  3 : Constant  Value=3
  4 : Constant  Value=4
  Add{,1..3} (4 alike) : Sum  Inputs=+-
  Enabled Subsystem1 : Subsystem  TreatAsAtomicUnit=on
  Enabled Subsystem2 : Subsystem  TreatAsAtomicUnit=on
  Enabled Subsystem3 : Subsystem  TreatAsAtomicUnit=on
  Enabled Subsystem4 : Subsystem  TreatAsAtomicUnit=on
  Mux2 : Mux
  disengahe : Constant  Value=-1
  engage : Constant
  selector{1..4} (4 alike) : Switch  Criteria=u2 ~= 0  Threshold=2300  ZeroCross=off
  Clutches : Outport
  wires:
  Mux2/1 -> Clutches/1
  engage/1 -> [engage]
  [disengage] -> selector1/1
  disengahe/1 -> [disengage]
  [engage] -> selector1/3
  control/1 -> Add/1, Add1/1, Add2/1, Add3/1
  Add/1 -> selector1/2
  1/1 -> Add/2
  [disengage] -> selector2/1
  [engage] -> selector2/3
  Add1/1 -> selector2/2
  2/1 -> Add1/2
  [disengage] -> selector3/1
  [engage] -> selector3/3
  Add2/1 -> selector3/2
  3/1 -> Add2/2
  [disengage] -> selector4/1
  [engage] -> selector4/3
  Add3/1 -> selector4/2
  4/1 -> Add3/2
  selector1/1 -> Enabled Subsystem1/Enable
  selector2/1 -> Enabled Subsystem2/Enable
  selector3/1 -> Enabled Subsystem3/Enable
  selector4/1 -> Enabled Subsystem4/Enable
  Enabled Subsystem1/1(clutch release) -> Mux2/1
  Enabled Subsystem2/1(clutch release) -> Mux2/2
  Enabled Subsystem3/1(clutch release) -> Mux2/3
  Enabled Subsystem4/1(clutch release) -> Mux2/4

== system hyd_hyb_2_int_cont_offline/hydraulic transmission/PM_hydraulic_machine /eta estimator/eta_t ==
  qv : Inport
  delta_p : Inport  Port=2
  Pmax : Inport  Port=3
  Abs : Abs
  Abs1 : Abs
  Constant : Constant  Value=600
  Constant1 : Constant  Value=0
  Divide : Product  Inputs=*/
  Product : Product  RndMeth=Zero
  Product1 : Product  RndMeth=Zero
  Saturation : Saturate  UpperLimit=1  LowerLimit=0
  Saturation1 : Saturate  UpperLimit=inf  LowerLimit=0.0000001
  Scope : Scope
      settings: SaveName=ScopeData29
  Scope1 : Scope  NumInputPorts=2
      settings: TimeRange=2.2  YMin=-5~-5  YMax=5~5  SaveName=ScopeData30
  Scope2 : Scope
      settings: YMin=0  YMax=190  SaveName=ScopeData50
  Scope3 : Scope
      settings: YMin=0  YMax=190  SaveName=ScopeData51
  Switch : Switch  Threshold=1
  eta_t : Outport
  wires:
  qv/1 -> Product1/1, Abs1/1
  delta_p/1 -> Product1/2
  Pmax/1 -> Product/1
  Constant/1 -> Product/2
  Product1/1 -> Abs/1
  Abs/1 -> Divide/1, Scope1/1
  Product/1 -> Saturation1/1
  Abs1/1 -> Scope2/1, Switch/2
  Saturation/1 -> eta_t/1
  Switch/1 -> Saturation/1, Scope/1
  Divide/1 -> Switch/1, Scope3/1
  Constant1/1 -> Switch/3
  Saturation1/1 -> Divide/2, Scope1/2

== system hyd_hyb_2_int_cont_offline/hydraulic transmission/PM_hydraulic_machine /eta estimator/eta_v ==
  qv : Inport
  vg : Inport  Port=2
  n : Inport  Port=3
  Abs : Abs
  Abs1 : Abs
  Abs2 : Abs
  Constant : Constant  Value=1000
  Constant1 : Constant  Value=0.00001
  Divide : Product  Inputs=*/
  Product : Product  RndMeth=Zero
  Product1 : Product  RndMeth=Zero
  Saturation : Saturate  UpperLimit=1  LowerLimit=0.000001
  Saturation1 : Saturate  UpperLimit=inf  LowerLimit=0.0000001
  Scope : Scope  NumInputPorts=2
      settings: TimeRange=2  YMin=-5~-5  YMax=5~5  SaveName=ScopeData43
  Scope1 : Scope
      settings: TimeRange=2  SaveName=ScopeData44
  Scope2 : Scope  NumInputPorts=2
      settings: TimeRange=2  YMin=-5~-5  YMax=5~5  SaveName=ScopeData45
  Scope3 : Scope  NumInputPorts=2
      settings: TimeRange=2  YMin=-5~-5  YMax=5~5  SaveName=ScopeData46
  Scope4 : Scope
      settings: SaveName=ScopeData52
  Switch : Switch  Threshold=1
  eta_v : Outport
  wires:
  n/1 -> Product/1, Scope2/1
  vg/1 -> Product/2, Scope2/2
  qv/1 -> Scope3/1, Product1/1, Abs2/1
  Constant/1 -> Product1/2
  Product1/1 -> Abs/1
  Abs/1 -> Divide/1, Scope/1
  Product/1 -> Abs1/1
  Abs1/1 -> Scope/2, Saturation1/1
  Divide/1 -> Switch/1, Scope4/1
  Constant1/1 -> Switch/3
  Switch/1 -> Saturation/1, Scope1/1
  Saturation/1 -> eta_v/1
  Abs2/1 -> Switch/2
  Saturation1/1 -> Divide/2

== system hyd_hyb_2_int_cont_offline/hydraulic transmission/accumulator/max - min volume estimator/for 10 gal accumulator ==
  min_press(psi) : Inport
  max_press(psi) : Inport  Port=2
  pre_ch_press(psi) : Inport  Port=3
  Action Port : ActionPort  PropagateVarSize=During execution  ActionType=then
  Constant : Constant  Value=152
  Scope : Scope  NumInputPorts=2
      settings: YMin=-5~-5  YMax=5~5  SaveName=ScopeData40
  Scope1 : Scope  NumInputPorts=2
      settings: YMin=-5~-5  YMax=5~5  SaveName=ScopeData41
  in^3 to lit : Gain  Gain=16.387e-3
  in^3 to lit (1) : Gain  Gain=16.387e-3
  rexroth-1 : Lookup_n-D  BreakpointsForDimension1=[1000,1100,1200,1300,1400,1500,1600,1700,1800,1900,2000,2100,2200,2300,2400,2500,2600,2700,2800,2900,3000,3100,3200,3300,3400,3500,3600,3700,3800,3900,4000,4100,4200,4300,4400,4500,4600,4700,4800,4900,5000,5100,5200,5300,5400,5500,5600,5700,5800,5900,6000]  BreakpointsForDimension2=[1000,1400,2000]  Table=v_p_10  InputSameDT=on
  rexroth-10 : Lookup_n-D  BreakpointsForDimension1=[1000,1100,1200,1300,1400,1500,1600,1700,1800,1900,2000,2100,2200,2300,2400,2500,2600,2700,2800,2900,3000,3100,3200,3300,3400,3500,3600,3700,3800,3900,4000,4100,4200,4300,4400,4500,4600,4700,4800,4900,5000,5100,5200,5300,5400,5500,5600,5700,5800,5900,6000]  BreakpointsForDimension2=[1000,1400,2000]  Table=v_p_10  InputSameDT=on
  min_vol(lit) : Outport
  max_vol(lit) : Outport  Port=2
  accum_dry_mass ( kg ) : Outport  Port=3  InitialOutput=[0]
  wires:
  in^3 to lit/1 -> min_vol(lit)/1, Scope1/1
  rexroth-10/1 -> in^3 to lit (1)/1, Scope/2
  rexroth-1/1 -> in^3 to lit/1, Scope/1
  in^3 to lit (1)/1 -> max_vol(lit)/1, Scope1/2
  pre_ch_press(psi)/1 -> rexroth-10/2, rexroth-1/2
  min_press(psi)/1 -> rexroth-1/1
  max_press(psi)/1 -> rexroth-10/1
  Constant/1 -> accum_dry_mass ( kg )/1

== system hyd_hyb_2_int_cont_offline/hydraulic transmission/accumulator/max - min volume estimator/for 15 gal accumulator1 ==
  min_press(psi) : Inport
  max_press(psi) : Inport  Port=2
  pre_ch_press(psi) : Inport  Port=3
  Action Port : ActionPort  PropagateVarSize=During execution  ActionType=then
  Constant : Constant  Value=220
  Scope : Scope  NumInputPorts=2
      settings: YMin=-5~-5  YMax=5~5  SaveName=ScopeData38
  Scope1 : Scope  NumInputPorts=2
      settings: YMin=4.74484~24.0403  YMax=4.74484~24.0403  SaveName=ScopeData39
  in^3 to lit : Gain  Gain=16.387e-3
  in^3 to lit (1) : Gain  Gain=16.387e-3
  rexroth-1 : Lookup_n-D  BreakpointsForDimension1=[1000,1100,1200,1300,1400,1500,1600,1700,1800,1900,2000,2100,2200,2300,2400,2500,2600,2700,2800,2900,3000,3100,3200,3300,3400,3500,3600,3700,3800,3900,4000,4100,4200,4300,4400,4500,4600,4700,4800,4900,5000,5100,5200,5300,5400,5500,5600,5700,5800,5900,6000]  BreakpointsForDimension2=[1000,1400,2000]  Table=v_p_15  InputSameDT=on
  rexroth-15 : Lookup_n-D  BreakpointsForDimension1=[1000,1100,1200,1300,1400,1500,1600,1700,1800,1900,2000,2100,2200,2300,2400,2500,2600,2700,2800,2900,3000,3100,3200,3300,3400,3500,3600,3700,3800,3900,4000,4100,4200,4300,4400,4500,4600,4700,4800,4900,5000,5100,5200,5300,5400,5500,5600,5700,5800,5900,6000]  BreakpointsForDimension2=[1000,1400,2000]  Table=v_p_15  InputSameDT=on
  min_vol(lit) : Outport
  max_vol(lit) : Outport  Port=2
  accum_dry_mass ( kg ) : Outport  Port=3  InitialOutput=[0]
  wires:
  in^3 to lit/1 -> min_vol(lit)/1, Scope1/1
  rexroth-1/1 -> in^3 to lit (1)/1, Scope/2
  rexroth-15/1 -> in^3 to lit/1, Scope/1
  in^3 to lit (1)/1 -> max_vol(lit)/1, Scope1/2
  pre_ch_press(psi)/1 -> rexroth-15/2, rexroth-1/2
  min_press(psi)/1 -> rexroth-15/1
  max_press(psi)/1 -> rexroth-1/1
  Constant/1 -> accum_dry_mass ( kg )/1
